simulink model "fxlms_s"  (R2016b)
settings: Solver=FixedStepDiscrete  StartTime=0.0  StopTime=inf  RelTol=1e-3  EnableMultiTasking=on
undefined symbols (not defined in the file or in its folder): SecondaryPath
libraries: dspvision x2, dspsnks4 x1, dspadpt3 x1, dspsrcs4 x1
settings Model: Creator=xiezh  LastModifiedBy=xiezh
settings SolverCC: ZeroCrossAlgorithm=Adaptive

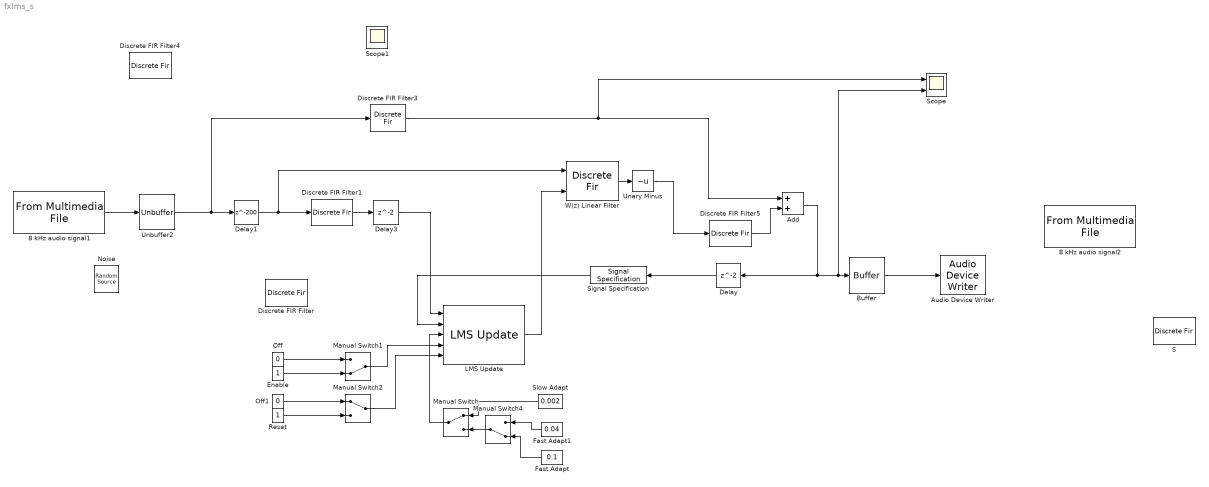
== system fxlms_s ==
  8 kHz audio signal1 : dspvision/From Multimedia File  inputFilename=C:\Users\xiezh\Documents\Signal&System\project\noise.wav  loop=on  numPlays=inf  outputStreams=Audio only  videoDataType=single  audioDataType=single  inheritSampleTime=off  userDefinedSampleTime=1/8000  noAudioOutput=off  isIntensityVideo=off  fourcc=RGB  colorVideoFormat=Separate color signals  outputEOF=off  dataOrg=Column-major  audioFrameSize=32  computeAudioFrameSize=off  outSamplingMode=Sample based
  8 kHz audio signal2 : dspvision/From Multimedia File  inputFilename=C:\Users\xiezh\Documents\Signal&System\project\noise.wav  loop=on  numPlays=inf  outputStreams=Audio only  videoDataType=single  audioDataType=single  inheritSampleTime=off  userDefinedSampleTime=1/8000  noAudioOutput=off  isIntensityVideo=off  fourcc=RGB  colorVideoFormat=Separate color signals  outputEOF=off  dataOrg=Column-major  audioFrameSize=32  computeAudioFrameSize=off  outSamplingMode=Sample based
  Add : Sum
  Audio Device Writer : dspsnks4/Audio Device Writer  Driver=ASIO  Device=ASIO4ALL v2  InheritSampleRate=off  SampleRate=8000  BitDepth=16-bit integer  BufferSize=4096  NumBuffers=10  DefaultOutputChannelMapping=on  OutputChannelMapping=1:2  OutputNumUnderrunSamples=off  DriverIdx=3  DeviceWarnFlag=''
  Buffer : Buffer  N=32  TreatMby1Signals=One channel  OutputFrames=off
  Delay : Delay
  Delay1 : Delay  DelayLength=200
  Delay3 : Delay
  Discrete FIR Filter : DiscreteFir  Coefficients=[1,1]
  Discrete FIR Filter1 : DiscreteFir  Coefficients=[.2,.3,.4]
  Discrete FIR Filter3 : DiscreteFir  Coefficients="[.9 .8 .7 .6 .5 .4 -0.0187632697069697\t0.0118916413750900\t0.0187632697069697\t-0.0118916413750900\t-0.0187632697069697\t0.0118916413750900\t0.0187632697069697\t-0.0118916413750900\t-0.0187632697069697\t0.0118916413750900\t0.0187632697069697\t-0.0118916413750900\t-0.0187632697069697\t0.0118916413750900\t0.0187632697069697\t-0.0118916413750900\t-0.0187632697069697\t0.0118916413750900\t0.0187632697069697\t-0.0118916413750900\t-0.0187632697069697\t0.0118916413750900\t0.0187632697069697\t-0.0118916413750900\t-0.0187632697069697\t0.0118916413750900\t0.0187632697069697\t-0.0118916413750900\t-0.0187632697069697\t0.0118916413750900\t0.0187632697069697\t-0.0118916413750900\t-0.0187632697069697\t0.0118993769403947\t0.0187676730001025\t-0.0119157086130632\t-0.0187727319443278\t0.0118975664493097\t0.0187643798434787\t-0.0118756654676450\t-0.0187267599993996\t0.0118686153557552\t0.0187441962206416\t-0.0118633254435314\t-0.0187353747332148\t0.0119006975558056\t0.0187459173047595\t-0.0118768910881532\t-0.0187290324264817\t0.0118699061688436\t0.0187251208716683\t-0.0118876068856968\t-0.0187225206190400\t0.0118946420964254\t0.0187421957397513\t-0.0118818885650886\t-0.0187472137057833\t0.0118771499958290\t0.0187150327855401\t-0.0118879421618236\t-0.0187069675320439\t0.0118853270080341\t0.0187100222700887\t-0.0118710479703201\t-0.0187251804763131\t0.0118719867434753\t0.0187058871978574\t-0.0118873926815046\t-0.0186986489588074\t0.0118873461153759\t0.0187052576237969\t-0.0118930998262418\t-0.0187001651519589\t0.0119098245170368\t0.0187102681392483\t-0.0119152336385502\t-0.0187214216584019\t0.0119162040766729\t0.0186924388998799\t-0.0119448254820360\t-0.0187187096470647\t0.0119146152403606\t0.0187211757892422\t-0.0119006305005802\t-0.0187120339268498\t0.0119112922814144\t0.0187231539183907\t-0.0118958882060302\t-0.0187112329894357\t0.0118957783099664\t0.0187134309107117\t-0.0118990975436224\t-0.0187254747742467\t0.0118775187995685\t0.0187119482451730\t-0.0118621761914743\t-0.0187035924190335\t0.0118837046441091\t0.0187172158056550\t-0.0118724747565044]"
  Discrete FIR Filter4 : DiscreteFir  Coefficients="[0.00222607343490954\t-0.00102528008164045\t0.00106052469338320\t-0.00154306873195859\t-0.00408800632849974\t0.00168928523190151\t0.000348074507221575\t0.00464509931112755\t-0.00283163308313110\t-0.000733294586663067\t-0.00404284345127758\t-0.00100898092243165\t-0.000879198417205976\t0.000415019617530972\t0.00177106295522287\t0.00417590443330956\t0.00171830143216876\t-0.000853900829708825\t-0.00553424934071462\t-0.00343464125874844\t0.00219100589321537\t0.000535164214723058\t0.00814873691495626\t-0.00123813190296196\t-0.00113693225111582\t-0.000762682264726267\t-0.000906980011165303\t-0.00101397255150104\t-0.000314435944149929\t0.000942960345591654\t0.00441021753715298\t-0.00410957052570594\t5.84253032347294e-05\t-0.00529636955227991\t0.00215281161466876\t0.000882325655660018\t0.000486138372037793\t-0.00297127062582664\t0.00604202964919128\t0.00422315436793293\t0.00136330161487315\t0.000917650151925748\t-0.00496073062156396\t-0.000352985068296105\t0.00176837659612645\t-0.00277365156764396\t-0.00533427499901304\t-0.00358083302015304\t-0.00591818394791430\t0.00552980550259345\t0.000628857816235480\t0.00797907798214535\t0.00289108015719185\t0.00618228108852445\t-0.00919985987552745\t-0.00449623653595545\t-0.000622126106680277\t0.00123691778158443\t0.00733060119151331\t-0.00680515679999299\t0.00647436259534561\t-0.0105561157197112\t-0.00268283746889520\t0.00146570760249302\t0.00663069442064955\t0.00179561862456719\t0.000401719790185424\t-0.00306260901242393\t-0.00212827929920107\t0.00180982854014213\t-0.00549750246673840\t0.00996985424448021\t-0.00336297072324468\t0.000180049704428702\t-9.85382078445304e-05]"
  Discrete FIR Filter5 : DiscreteFir  Coefficients=[.2,.3,.4]
  Enable : Constant  OutDataTypeStr=boolean
  Fast Adapt : Constant  Value=0.1  OutDataTypeStr=single
  Fast Adapt1 : Constant  Value=0.04  OutDataTypeStr=single
  LMS Update : dspadpt3/LMS Update  Method=Normalized LMS  Length=100  StepSizeSource=Input port  StepSize=0.1  LeakageFactor=1.0  InitialConditions=0  EnableAdaptInput=on  EnableResetInput=on  SimulateUsing=Code generation
  Manual Switch : ManualSwitch
  Manual Switch1 : ManualSwitch  CurrentSetting=0
  Manual Switch2 : ManualSwitch
  Manual Switch4 : ManualSwitch  CurrentSetting=0
  Noise : dspsrcs4/Random Source  SrcType=Gaussian  NormMethod=Sum of uniform values  CltLength=5  MinVal=-1  MaxVal=1  MeanVal=0  VarVal=1  RepMode=Specify seed  rawSeed=[23341]  IsInherit=off  SampMode=Discrete  SampTime=1/8000  SampFrame=2  DataType=Single  OutComplex=Real  OutputFrames=off
  Off : Constant  Value=0  OutDataTypeStr=boolean
  Off1 : Constant  Value=0  OutDataTypeStr=boolean
  Reset : Constant  OutDataTypeStr=boolean
  "S " : DiscreteFir  Coefficients="[-0.00115293973549078\t0.000521845152236082\t0.00129424555693093\t0.000467902429182095\t-0.000399698413473190\t-0.00175454756738187\t-0.000741983536064869\t0.00195925902669584\t0.00257037269003199\t-0.00160732757728425\t-0.00130653905245927\t0.000330533835821434\t-0.000668810246848779\t0.00123739234321625\t6.02462844603704e-05\t-0.00180028576027474\t-0.000890457813617406\t0.000684745236926885\t0.00166523368052551\t0.000304441218749564\t0.000459335667653556\t-0.000981302364080229\t0.000188139447255483\t0.000214983577451476\t-0.000952475530175957\t0.000987305255910752\t0.000363014541547280\t-0.00145229186428641\t-0.00179987998108309\t0.00223084297863409\t0.00205395101762280\t0.00102152915995323\t0.000798470882593062\t-0.00349544765435155\t-0.00265039741946524\t-2.86827230734000e-05\t0.00193822327182870\t0.000985296515478774\t-9.39562796562895e-05\t0.00163654303797938\t0.000380660152911000\t-0.000316497642702500\t-0.00294636344555872\t-0.00128818191787820\t-0.00166826567529997\t0.000797982138240058\t0.00191512845646011\t-0.000177068650519784\t0.00266804122382235\t0.00120196959116323\t-0.00177506044202936\t-0.00100313952482596\t-0.00170733332509806\t0.000360859976225875\t0.00192332205348316\t-0.00128508511426898\t0.000398724444984378\t-0.000975482439971784\t-0.00204407314541213\t0.00355543818648772\t0.00118670995366865\t-0.000552447728129918\t0.00167750222636686\t-0.00104445587591862\t-0.00170375845005344\t-0.00135467881437353\t0.00133495609664194\t0.00113880591795151\t-0.000969131941962797\t-0.000787423383126802\t-0.00101406913377130\t0.000228551982551214\t-0.000395248066108801\t0.000343931545560962\t0.000416862678532092]"  InputProcessing=Columns as channels (frame based)
  Scope : Scope  NumInputPorts=2
  Signal Specification : SignalSpecification  OutDataTypeStr=single  Dimensions=[1 1]
      settings: LockScale=on
  Slow Adapt : Constant  Value=0.002  OutDataTypeStr=single
  Unary Minus : UnaryMinus
  Unbuffer2 : Unbuffer  SampleBasedProcessing=Same as frame based
  W(z) Linear Filter : DiscreteFir  CoefSource=Input port  Coefficients=SecondaryPath  AccumDataTypeStr=Inherit: Same as product output  OutDataTypeStr=Inherit: Same as input
      settings: InputPortMap=u0,u1  LockScale=on
  Scope1 : Scope
  wires:
  Off/1 -> Manual Switch1/1
  Enable/1 -> Manual Switch1/2
  Off1/1 -> Manual Switch2/1
  Reset/1 -> Manual Switch2/2
  Slow Adapt/1 -> Manual Switch/1
  Manual Switch4/1 -> Manual Switch/2
  Fast Adapt1/1 -> Manual Switch4/1
  Fast Adapt/1 -> Manual Switch4/2
  Manual Switch2/1 -> LMS Update/5
  Manual Switch1/1 -> LMS Update/4
  Manual Switch/1 -> LMS Update/3
  W(z) Linear Filter/1 -> Unary Minus/1
  Signal Specification/1 -> LMS Update/2
  LMS Update/1 -> W(z) Linear Filter/2
  Buffer/1 -> Audio Device Writer/1
  8 kHz audio signal1/1 -> Unbuffer2/1
  Add/1 -> Delay/1, Scope/2, Buffer/1
  Delay/1 -> Signal Specification/1
  Discrete FIR Filter5/1 -> Add/2
  Discrete FIR Filter3/1 -> Scope/1, Add/1
  Delay3/1 -> LMS Update/1
  Unary Minus/1 -> Discrete FIR Filter5/1
  Discrete FIR Filter1/1 -> Delay3/1
  Unbuffer2/1 -> Delay1/1, Discrete FIR Filter3/1
  Delay1/1 -> Discrete FIR Filter1/1, W(z) Linear Filter/1
